simulink model "kif_halozat"  (R2020a)
settings: Solver=VariableStepAuto  StartTime=0.0  StopTime=10.0  RelTol=1e-3
libraries: powerlib x95, ee_lib x33
settings Model: Creator=Ákos  LastModifiedBy=Ákos

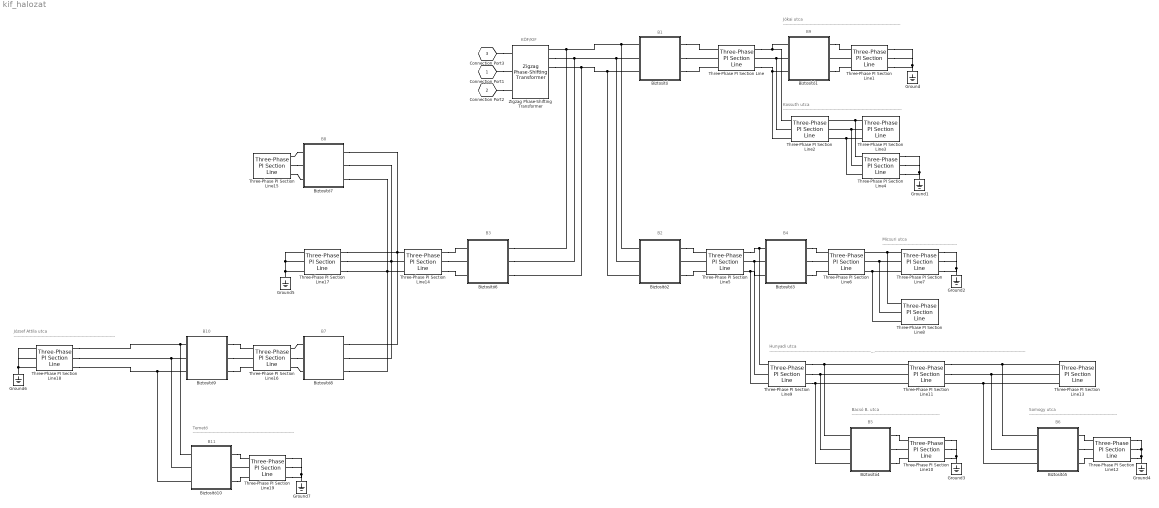
== system kif_halozat ==
  note: B2
  note: Jókai utca
      | ----------------------------------------------------------------------------------------
  note: B9
  note: B1
  note: KÖF/KIF
  note: Kossuth utca
      | -----------------------------------------------------------------------------------------
  note: B4
  note: Micsuri utca
      | --------------------------------------------------------
  note: B5
  note: B6
  note: Bacsó B. utca
      | ------------------------------------------------------------------
  note: Somogy utca
      | ------------------------------------------------------------------
  note: Hunyadi utca
      | -----------------------------------------------------------------------------------------------------------------------------------------------------------------------------------------------------------------------
  note: B3
  note: B8
  note: B7
  note: B10
  note: József Attila utca
      | ----------------------------------------------------------------------------
  note: B11
  note: Temető
      | ----------------------------------------------------------------------------
  Biztosító : Subsystem
  Biztosító1 : Subsystem
  Biztosító10 : Subsystem
  Biztosító2 : Subsystem
  Biztosító3 : Subsystem
  Biztosító4 : Subsystem
  Biztosító5 : Subsystem
  Biztosító6 : Subsystem
  Biztosító7 : Subsystem
  Biztosító8 : Subsystem
  Biztosító9 : Subsystem
  Ground{,1..7} (8 alike) : powerlib/Elements/Ground  LConnTagsString=a
  Three-Phase PI Section Line : powerlib/Elements/Three-Phase PI Section Line  LConnTagsString=a|b|c  RConnTagsString=A|B|C  Frequency=50  Resistances=[ 0.01273 0.3864]  Inductances="[ 0.9337e-3  4.1264e-3]"  Capacitances=[12.74e-9 7.751e-9]  Length=0.195
  Three-Phase PI Section Line1 : powerlib/Elements/Three-Phase PI Section Line  LConnTagsString=a|b|c  RConnTagsString=A|B|C  Frequency=50  Resistances=[ 0.01273 0.3864]  Inductances="[ 0.9337e-3  4.1264e-3]"  Capacitances=[12.74e-9 7.751e-9]  Length=0.3
  Three-Phase PI Section Line10 : powerlib/Elements/Three-Phase PI Section Line  LConnTagsString=a|b|c  RConnTagsString=A|B|C  Frequency=50  Resistances=[ 0.01273 0.3864]  Inductances="[ 0.9337e-3  4.1264e-3]"  Capacitances=[12.74e-9 7.751e-9]  Length=0.193
  Three-Phase PI Section Line11 : powerlib/Elements/Three-Phase PI Section Line  LConnTagsString=a|b|c  RConnTagsString=A|B|C  Frequency=50  Resistances=[ 0.01273 0.3864]  Inductances="[ 0.9337e-3  4.1264e-3]"  Capacitances=[12.74e-9 7.751e-9]  Length=0.151
  Three-Phase PI Section Line12 : powerlib/Elements/Three-Phase PI Section Line  LConnTagsString=a|b|c  RConnTagsString=A|B|C  Frequency=50  Resistances=[ 0.01273 0.3864]  Inductances="[ 0.9337e-3  4.1264e-3]"  Capacitances=[12.74e-9 7.751e-9]  Length=0.151
  Three-Phase PI Section Line13 : powerlib/Elements/Three-Phase PI Section Line  LConnTagsString=a|b|c  RConnTagsString=A|B|C  Frequency=50  Resistances=[ 0.01273 0.3864]  Inductances="[ 0.9337e-3  4.1264e-3]"  Capacitances=[12.74e-9 7.751e-9]  Length=0.151
  Three-Phase PI Section Line14 : powerlib/Elements/Three-Phase PI Section Line  LConnTagsString=a|b|c  RConnTagsString=A|B|C  Frequency=50  Resistances=[ 0.01273 0.3864]  Inductances="[ 0.9337e-3  4.1264e-3]"  Capacitances=[12.74e-9 7.751e-9]  Length=0.063
  Three-Phase PI Section Line15 : powerlib/Elements/Three-Phase PI Section Line  LConnTagsString=a|b|c  RConnTagsString=A|B|C  Frequency=50  Resistances=[ 0.01273 0.3864]  Inductances="[ 0.9337e-3  4.1264e-3]"  Capacitances=[12.74e-9 7.751e-9]  Length=0.010
  Three-Phase PI Section Line16 : powerlib/Elements/Three-Phase PI Section Line  LConnTagsString=a|b|c  RConnTagsString=A|B|C  Frequency=50  Resistances=[ 0.01273 0.3864]  Inductances="[ 0.9337e-3  4.1264e-3]"  Capacitances=[12.74e-9 7.751e-9]  Length=0.249
  Three-Phase PI Section Line17 : powerlib/Elements/Three-Phase PI Section Line  LConnTagsString=a|b|c  RConnTagsString=A|B|C  Frequency=50  Resistances=[ 0.01273 0.3864]  Inductances="[ 0.9337e-3  4.1264e-3]"  Capacitances=[12.74e-9 7.751e-9]  Length=0.217
  Three-Phase PI Section Line18 : powerlib/Elements/Three-Phase PI Section Line  LConnTagsString=a|b|c  RConnTagsString=A|B|C  Frequency=50  Resistances=[ 0.01273 0.3864]  Inductances="[ 0.9337e-3  4.1264e-3]"  Capacitances=[12.74e-9 7.751e-9]  Length=0.157
  Three-Phase PI Section Line19 : powerlib/Elements/Three-Phase PI Section Line  LConnTagsString=a|b|c  RConnTagsString=A|B|C  Frequency=50  Resistances=[ 0.01273 0.3864]  Inductances="[ 0.9337e-3  4.1264e-3]"  Capacitances=[12.74e-9 7.751e-9]  Length=0.187
  Three-Phase PI Section Line2 : powerlib/Elements/Three-Phase PI Section Line  LConnTagsString=a|b|c  RConnTagsString=A|B|C  Frequency=50  Resistances=[ 0.01273 0.3864]  Inductances="[ 0.9337e-3  4.1264e-3]"  Capacitances=[12.74e-9 7.751e-9]  Length=0.317
  Three-Phase PI Section Line3 : powerlib/Elements/Three-Phase PI Section Line  LConnTagsString=a|b|c  RConnTagsString=A|B|C  Frequency=50  Resistances=[ 0.01273 0.3864]  Inductances="[ 0.9337e-3  4.1264e-3]"  Capacitances=[12.74e-9 7.751e-9]  Length=0.078
  Three-Phase PI Section Line4 : powerlib/Elements/Three-Phase PI Section Line  LConnTagsString=a|b|c  RConnTagsString=A|B|C  Frequency=50  Resistances=[ 0.01273 0.3864]  Inductances="[ 0.9337e-3  4.1264e-3]"  Capacitances=[12.74e-9 7.751e-9]  Length=0.036
  Three-Phase PI Section Line5 : powerlib/Elements/Three-Phase PI Section Line  LConnTagsString=a|b|c  RConnTagsString=A|B|C  Frequency=50  Resistances=[ 0.01273 0.3864]  Inductances="[ 0.9337e-3  4.1264e-3]"  Capacitances=[12.74e-9 7.751e-9]  Length=0.070
  Three-Phase PI Section Line6 : powerlib/Elements/Three-Phase PI Section Line  LConnTagsString=a|b|c  RConnTagsString=A|B|C  Frequency=50  Resistances=[ 0.01273 0.3864]  Inductances="[ 0.9337e-3  4.1264e-3]"  Capacitances=[12.74e-9 7.751e-9]  Length=0.092
  Three-Phase PI Section Line7 : powerlib/Elements/Three-Phase PI Section Line  LConnTagsString=a|b|c  RConnTagsString=A|B|C  Frequency=50  Resistances=[ 0.01273 0.3864]  Inductances="[ 0.9337e-3  4.1264e-3]"  Capacitances=[12.74e-9 7.751e-9]  Length=0.270
  Three-Phase PI Section Line8 : powerlib/Elements/Three-Phase PI Section Line  LConnTagsString=a|b|c  RConnTagsString=A|B|C  Frequency=50  Resistances=[ 0.01273 0.3864]  Inductances="[ 0.9337e-3  4.1264e-3]"  Capacitances=[12.74e-9 7.751e-9]  Length=0.066
  Three-Phase PI Section Line9 : powerlib/Elements/Three-Phase PI Section Line  LConnTagsString=a|b|c  RConnTagsString=A|B|C  Frequency=50  Resistances=[ 0.01273 0.3864]  Inductances="[ 0.9337e-3  4.1264e-3]"  Capacitances=[12.74e-9 7.751e-9]  Length=0.106
  Zigzag Phase-Shifting Transformer : powerlib/Elements/Zigzag Phase-Shifting Transformer  SecondaryConnection=Y  SetSaturation=off  SetInitialFlux=off  Measurements=None  UNITS=SI  NominalPower=[ 120e3 50]  PrimaryVoltage=0.42e3  SecondaryVoltage="[ 21e3  +90]"  Winding1=[0.002488 0.00026399]  Winding2=[0.00017863 1.8954e-05]  Winding3=[0.018 0.0019099]  RmLm=[622.01 1.6499]  Rm=622.01  Saturation=[0 0;17.569 28.988;7320.5 36.718]  InitialFluxes=[0 0 0]  BreakLoop=off  DiscreteSolver=Trapezoidal iterative  DataType=on
      settings: SourceProductBaseCode=PS
  Connection Port1 : PMIOPort  Tag=PMCPort  Side=Left
  Connection Port2 : PMIOPort  Tag=PMCPort  Port=2  Side=Left
  Connection Port3 : PMIOPort  Tag=PMCPort  Port=3  Side=Left
  connections:
  Biztosító/RConn1 -- Three-Phase PI Section Line/LConn1
  Biztosító/LConn1 -- Biztosító2/LConn1 -- Biztosító6/LConn1 -- Zigzag Phase-Shifting Transformer/LConn1
  Biztosító/RConn2 -- Three-Phase PI Section Line/LConn2
  Zigzag Phase-Shifting Transformer/LConn2 -- Biztosító6/LConn2 -- Biztosító2/LConn2 -- Biztosító/LConn2
  Biztosító/RConn3 -- Three-Phase PI Section Line/LConn3
  Zigzag Phase-Shifting Transformer/LConn3 -- Biztosító6/LConn3 -- Biztosító2/LConn3 -- Biztosító/LConn3
  Biztosító1/LConn2 -- Three-Phase PI Section Line2/LConn2 -- Three-Phase PI Section Line/RConn2
  Three-Phase PI Section Line/RConn1 -- Three-Phase PI Section Line2/LConn1 -- Biztosító1/LConn1
  Three-Phase PI Section Line/RConn3 -- Three-Phase PI Section Line2/LConn3 -- Biztosító1/LConn3
  Three-Phase PI Section Line1/LConn2 -- Biztosító1/RConn2
  Biztosító1/RConn1 -- Three-Phase PI Section Line1/LConn1
  Biztosító1/RConn3 -- Three-Phase PI Section Line1/LConn3
  Three-Phase PI Section Line1/RConn3 -- Three-Phase PI Section Line1/RConn1 -- Three-Phase PI Section Line1/RConn2 -- Ground/LConn1
  Three-Phase PI Section Line3/LConn1 -- Three-Phase PI Section Line4/LConn1 -- Three-Phase PI Section Line2/RConn1
  Three-Phase PI Section Line3/LConn2 -- Three-Phase PI Section Line4/LConn2 -- Three-Phase PI Section Line2/RConn2
  Three-Phase PI Section Line3/LConn3 -- Three-Phase PI Section Line4/LConn3 -- Three-Phase PI Section Line2/RConn3
  Three-Phase PI Section Line4/RConn1 -- Three-Phase PI Section Line4/RConn2 -- Three-Phase PI Section Line4/RConn3 -- Ground1/LConn1
  Three-Phase PI Section Line5/LConn2 -- Biztosító2/RConn2
  Biztosító2/RConn1 -- Three-Phase PI Section Line5/LConn1
  Biztosító2/RConn3 -- Three-Phase PI Section Line5/LConn3
  Biztosító3/LConn2 -- Three-Phase PI Section Line9/LConn2 -- Three-Phase PI Section Line5/RConn2
  Three-Phase PI Section Line5/RConn1 -- Three-Phase PI Section Line9/LConn1 -- Biztosító3/LConn1
  Three-Phase PI Section Line5/RConn3 -- Three-Phase PI Section Line9/LConn3 -- Biztosító3/LConn3
  Biztosító3/RConn1 -- Three-Phase PI Section Line6/LConn1
  Biztosító3/RConn2 -- Three-Phase PI Section Line6/LConn2
  Biztosító3/RConn3 -- Three-Phase PI Section Line6/LConn3
  Three-Phase PI Section Line7/LConn1 -- Three-Phase PI Section Line8/LConn1 -- Three-Phase PI Section Line6/RConn1
  Three-Phase PI Section Line7/LConn2 -- Three-Phase PI Section Line8/LConn2 -- Three-Phase PI Section Line6/RConn2
  Three-Phase PI Section Line7/LConn3 -- Three-Phase PI Section Line8/LConn3 -- Three-Phase PI Section Line6/RConn3
  Ground2/LConn1 -- Three-Phase PI Section Line7/RConn3 -- Three-Phase PI Section Line7/RConn1 -- Three-Phase PI Section Line7/RConn2
  Three-Phase PI Section Line9/RConn1 -- Three-Phase PI Section Line11/LConn1 -- Biztosító4/LConn1
  Three-Phase PI Section Line9/RConn2 -- Three-Phase PI Section Line11/LConn2 -- Biztosító4/LConn2
  Three-Phase PI Section Line9/RConn3 -- Three-Phase PI Section Line11/LConn3 -- Biztosító4/LConn3
  Biztosító4/RConn1 -- Three-Phase PI Section Line10/LConn1
  Biztosító4/RConn2 -- Three-Phase PI Section Line10/LConn2
  Biztosító4/RConn3 -- Three-Phase PI Section Line10/LConn3
  Ground3/LConn1 -- Three-Phase PI Section Line10/RConn3 -- Three-Phase PI Section Line10/RConn1 -- Three-Phase PI Section Line10/RConn2
  Three-Phase PI Section Line11/RConn1 -- Three-Phase PI Section Line13/LConn1 -- Biztosító5/LConn1
  Three-Phase PI Section Line11/RConn2 -- Three-Phase PI Section Line13/LConn2 -- Biztosító5/LConn2
  Biztosító5/LConn3 -- Three-Phase PI Section Line13/LConn3 -- Three-Phase PI Section Line11/RConn3
  Three-Phase PI Section Line12/RConn1 -- Three-Phase PI Section Line12/RConn2 -- Three-Phase PI Section Line12/RConn3 -- Ground4/LConn1
  Biztosító5/RConn3 -- Three-Phase PI Section Line12/LConn3
  Biztosító5/RConn2 -- Three-Phase PI Section Line12/LConn2
  Biztosító5/RConn1 -- Three-Phase PI Section Line12/LConn1
  Three-Phase PI Section Line14/RConn1 -- Biztosító6/RConn1
  Three-Phase PI Section Line14/RConn2 -- Biztosító6/RConn2
  Three-Phase PI Section Line14/RConn3 -- Biztosító6/RConn3
  Biztosító7/RConn1 -- Three-Phase PI Section Line15/RConn1
  Three-Phase PI Section Line15/RConn2 -- Biztosító7/RConn2
  Three-Phase PI Section Line15/RConn3 -- Biztosító7/RConn3
  Three-Phase PI Section Line16/RConn3 -- Biztosító8/RConn3
  Three-Phase PI Section Line16/RConn2 -- Biztosító8/RConn2
  Biztosító8/RConn1 -- Three-Phase PI Section Line16/RConn1
  Three-Phase PI Section Line17/RConn1 -- Biztosító8/LConn1 -- Biztosító7/LConn1 -- Three-Phase PI Section Line14/LConn1
  Three-Phase PI Section Line17/RConn2 -- Biztosító8/LConn2 -- Biztosító7/LConn2 -- Three-Phase PI Section Line14/LConn2
  Three-Phase PI Section Line17/RConn3 -- Biztosító8/LConn3 -- Biztosító7/LConn3 -- Three-Phase PI Section Line14/LConn3
  Three-Phase PI Section Line17/LConn1 -- Three-Phase PI Section Line17/LConn2 -- Three-Phase PI Section Line17/LConn3 -- Ground5/LConn1
  Biztosító9/LConn2 -- Three-Phase PI Section Line16/LConn2
  Biztosító9/LConn1 -- Three-Phase PI Section Line16/LConn1
  Biztosító9/LConn3 -- Three-Phase PI Section Line16/LConn3
  Three-Phase PI Section Line18/LConn3 -- Three-Phase PI Section Line18/LConn1 -- Three-Phase PI Section Line18/LConn2 -- Ground6/LConn1
  Three-Phase PI Section Line18/RConn2 -- Biztosító10/LConn2 -- Biztosító9/RConn2
  Three-Phase PI Section Line18/RConn1 -- Biztosító10/LConn1 -- Biztosító9/RConn1
  Three-Phase PI Section Line18/RConn3 -- Biztosító10/LConn3 -- Biztosító9/RConn3
  Three-Phase PI Section Line19/LConn2 -- Biztosító10/RConn2
  Biztosító10/RConn1 -- Three-Phase PI Section Line19/LConn1
  Biztosító10/RConn3 -- Three-Phase PI Section Line19/LConn3
  Three-Phase PI Section Line19/RConn1 -- Three-Phase PI Section Line19/RConn2 -- Three-Phase PI Section Line19/RConn3 -- Ground7/LConn1
  Connection Port1/RConn1 -- Zigzag Phase-Shifting Transformer/RConn2
  Connection Port2/RConn1 -- Zigzag Phase-Shifting Transformer/RConn3
  Connection Port3/RConn1 -- Zigzag Phase-Shifting Transformer/RConn1

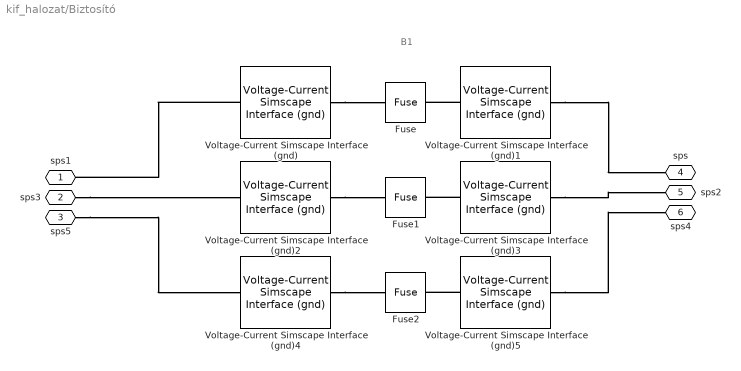
== system kif_halozat/Biztosító ==
  note: B1
  Fuse : ee_lib/Switches & Breakers/Fuse  prm=1  I_rated=125 A  melt_margin=1  T_fuse=0 s  I2t=1 s*A^2  I_vec=[1.9, 2, 2.5, 30] A  t_vec=[10000, 1, .3, .001] s  R_closed=0.01 Ohm  G_open=1e-8 1/Ohm  exposemeasurement=ee.enum.exposemeasurement.hidden
      settings: SourceProductBaseCode=PS  InternalSimscapePortConfiguration="{\"Bottom\":[],\"Left\":[{\"id\":\"p\",\"label\":\"\",\"type\":\"foundation.electrical.electrical\"}],\"Right\":[{\"id\":\"n\",\"label\":\"\",\"type\":\"foundation.electrical.electrical\"}],\"Top\":[]}"
  Fuse1 : ee_lib/Switches & Breakers/Fuse  prm=1  I_rated=125 A  melt_margin=1  T_fuse=0 s  I2t=1 s*A^2  I_vec=[1.9, 2, 2.5, 30] A  t_vec=[10000, 1, .3, .001] s  R_closed=0.01 Ohm  G_open=1e-8 1/Ohm  exposemeasurement=ee.enum.exposemeasurement.hidden
      settings: SourceProductBaseCode=PS  InternalSimscapePortConfiguration="{\"Bottom\":[],\"Left\":[{\"id\":\"p\",\"label\":\"\",\"type\":\"foundation.electrical.electrical\"}],\"Right\":[{\"id\":\"n\",\"label\":\"\",\"type\":\"foundation.electrical.electrical\"}],\"Top\":[]}"
  Fuse2 : ee_lib/Switches & Breakers/Fuse  prm=1  I_rated=125 A  melt_margin=1  T_fuse=0 s  I2t=1 s*A^2  I_vec=[1.9, 2, 2.5, 30] A  t_vec=[10000, 1, .3, .001] s  R_closed=0.01 Ohm  G_open=1e-8 1/Ohm  exposemeasurement=ee.enum.exposemeasurement.hidden
      settings: SourceProductBaseCode=PS  InternalSimscapePortConfiguration="{\"Bottom\":[],\"Left\":[{\"id\":\"p\",\"label\":\"\",\"type\":\"foundation.electrical.electrical\"}],\"Right\":[{\"id\":\"n\",\"label\":\"\",\"type\":\"foundation.electrical.electrical\"}],\"Top\":[]}"
  Voltage-Current Simscape Interface (gnd){,1..5} (6 alike) : powerlib/Interface Elements/Voltage-Current Simscape Interface (gnd)  DFT=off  Fmode=Low pass filter (continuous)  T=1e-6  Ts=50e-6  i0=0  v0=0  Sd=Specialized Power Systems side  Measurements=off
      settings: SourceProductBaseCode=PS
  sps1 : PMIOPort  Side=Left
  sps3 : PMIOPort  Port=2  Side=Left
  sps5 : PMIOPort  Port=3  Side=Left
  sps : PMIOPort  Port=4  Side=Right
  sps2 : PMIOPort  Port=5  Side=Right
  sps4 : PMIOPort  Port=6  Side=Right
  connections:
  Voltage-Current Simscape Interface (gnd)5/RConn1 -- Fuse2/RConn1
  Voltage-Current Simscape Interface (gnd)4/RConn1 -- Fuse2/LConn1
  sps3/RConn1 -- Voltage-Current Simscape Interface (gnd)2/LConn1
  Voltage-Current Simscape Interface (gnd)/RConn1 -- Fuse/LConn1
  Voltage-Current Simscape Interface (gnd)/LConn1 -- sps1/RConn1
  Voltage-Current Simscape Interface (gnd)1/RConn1 -- Fuse/RConn1
  Voltage-Current Simscape Interface (gnd)2/RConn1 -- Fuse1/LConn1
  sps5/RConn1 -- Voltage-Current Simscape Interface (gnd)4/LConn1
  Voltage-Current Simscape Interface (gnd)5/LConn1 -- sps4/RConn1
  Voltage-Current Simscape Interface (gnd)3/RConn1 -- Fuse1/RConn1
  Voltage-Current Simscape Interface (gnd)1/LConn1 -- sps/RConn1
  Voltage-Current Simscape Interface (gnd)3/LConn1 -- sps2/RConn1

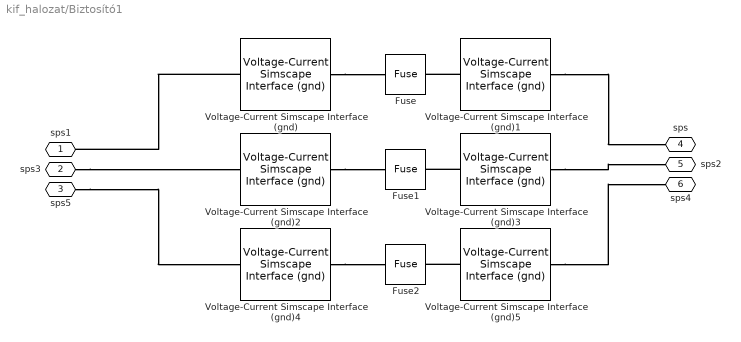
== system kif_halozat/Biztosító1 ==
  Fuse : ee_lib/Switches & Breakers/Fuse  prm=1  I_rated=80 A  melt_margin=1  T_fuse=0 s  I2t=1 s*A^2  I_vec=[1.9, 2, 2.5, 30] A  t_vec=[10000, 1, .3, .001] s  R_closed=0.01 Ohm  G_open=1e-8 1/Ohm  exposemeasurement=ee.enum.exposemeasurement.hidden
      settings: SourceProductBaseCode=PS  InternalSimscapePortConfiguration="{\"Bottom\":[],\"Left\":[{\"id\":\"p\",\"label\":\"\",\"type\":\"foundation.electrical.electrical\"}],\"Right\":[{\"id\":\"n\",\"label\":\"\",\"type\":\"foundation.electrical.electrical\"}],\"Top\":[]}"
  Fuse1 : ee_lib/Switches & Breakers/Fuse  prm=1  I_rated=80 A  melt_margin=1  T_fuse=0 s  I2t=1 s*A^2  I_vec=[1.9, 2, 2.5, 30] A  t_vec=[10000, 1, .3, .001] s  R_closed=0.01 Ohm  G_open=1e-8 1/Ohm  exposemeasurement=ee.enum.exposemeasurement.hidden
      settings: SourceProductBaseCode=PS  InternalSimscapePortConfiguration="{\"Bottom\":[],\"Left\":[{\"id\":\"p\",\"label\":\"\",\"type\":\"foundation.electrical.electrical\"}],\"Right\":[{\"id\":\"n\",\"label\":\"\",\"type\":\"foundation.electrical.electrical\"}],\"Top\":[]}"
  Fuse2 : ee_lib/Switches & Breakers/Fuse  prm=1  I_rated=80 A  melt_margin=1  T_fuse=0 s  I2t=1 s*A^2  I_vec=[1.9, 2, 2.5, 30] A  t_vec=[10000, 1, .3, .001] s  R_closed=0.01 Ohm  G_open=1e-8 1/Ohm  exposemeasurement=ee.enum.exposemeasurement.hidden
      settings: SourceProductBaseCode=PS  InternalSimscapePortConfiguration="{\"Bottom\":[],\"Left\":[{\"id\":\"p\",\"label\":\"\",\"type\":\"foundation.electrical.electrical\"}],\"Right\":[{\"id\":\"n\",\"label\":\"\",\"type\":\"foundation.electrical.electrical\"}],\"Top\":[]}"
  Voltage-Current Simscape Interface (gnd){,1..5} (6 alike) : powerlib/Interface Elements/Voltage-Current Simscape Interface (gnd)  DFT=off  Fmode=Low pass filter (continuous)  T=1e-6  Ts=50e-6  i0=0  v0=0  Sd=Specialized Power Systems side  Measurements=off
      settings: SourceProductBaseCode=PS
  sps1 : PMIOPort  Side=Left
  sps3 : PMIOPort  Port=2  Side=Left
  sps5 : PMIOPort  Port=3  Side=Left
  sps : PMIOPort  Port=4  Side=Right
  sps2 : PMIOPort  Port=5  Side=Right
  sps4 : PMIOPort  Port=6  Side=Right
  connections:
  Voltage-Current Simscape Interface (gnd)3/LConn1 -- sps2/RConn1
  Voltage-Current Simscape Interface (gnd)1/LConn1 -- sps/RConn1
  Voltage-Current Simscape Interface (gnd)3/RConn1 -- Fuse1/RConn1
  Voltage-Current Simscape Interface (gnd)5/LConn1 -- sps4/RConn1
  sps5/RConn1 -- Voltage-Current Simscape Interface (gnd)4/LConn1
  Voltage-Current Simscape Interface (gnd)2/RConn1 -- Fuse1/LConn1
  Voltage-Current Simscape Interface (gnd)1/RConn1 -- Fuse/RConn1
  Voltage-Current Simscape Interface (gnd)/LConn1 -- sps1/RConn1
  Voltage-Current Simscape Interface (gnd)/RConn1 -- Fuse/LConn1
  sps3/RConn1 -- Voltage-Current Simscape Interface (gnd)2/LConn1
  Voltage-Current Simscape Interface (gnd)4/RConn1 -- Fuse2/LConn1
  Voltage-Current Simscape Interface (gnd)5/RConn1 -- Fuse2/RConn1

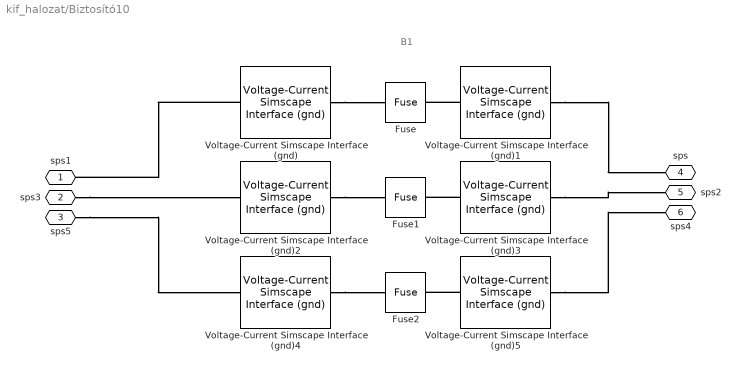
== system kif_halozat/Biztosító10 ==
  note: B1
  Fuse : ee_lib/Switches & Breakers/Fuse  prm=1  I_rated=125 A  melt_margin=1  T_fuse=0 s  I2t=1 s*A^2  I_vec=[1.9, 2, 2.5, 30] A  t_vec=[10000, 1, .3, .001] s  R_closed=0.01 Ohm  G_open=1e-8 1/Ohm  exposemeasurement=ee.enum.exposemeasurement.hidden
      settings: SourceProductBaseCode=PS  InternalSimscapePortConfiguration="{\"Bottom\":[],\"Left\":[{\"id\":\"p\",\"label\":\"\",\"type\":\"foundation.electrical.electrical\"}],\"Right\":[{\"id\":\"n\",\"label\":\"\",\"type\":\"foundation.electrical.electrical\"}],\"Top\":[]}"
  Fuse1 : ee_lib/Switches & Breakers/Fuse  prm=1  I_rated=125 A  melt_margin=1  T_fuse=0 s  I2t=1 s*A^2  I_vec=[1.9, 2, 2.5, 30] A  t_vec=[10000, 1, .3, .001] s  R_closed=0.01 Ohm  G_open=1e-8 1/Ohm  exposemeasurement=ee.enum.exposemeasurement.hidden
      settings: SourceProductBaseCode=PS  InternalSimscapePortConfiguration="{\"Bottom\":[],\"Left\":[{\"id\":\"p\",\"label\":\"\",\"type\":\"foundation.electrical.electrical\"}],\"Right\":[{\"id\":\"n\",\"label\":\"\",\"type\":\"foundation.electrical.electrical\"}],\"Top\":[]}"
  Fuse2 : ee_lib/Switches & Breakers/Fuse  prm=1  I_rated=125 A  melt_margin=1  T_fuse=0 s  I2t=1 s*A^2  I_vec=[1.9, 2, 2.5, 30] A  t_vec=[10000, 1, .3, .001] s  R_closed=0.01 Ohm  G_open=1e-8 1/Ohm  exposemeasurement=ee.enum.exposemeasurement.hidden
      settings: SourceProductBaseCode=PS  InternalSimscapePortConfiguration="{\"Bottom\":[],\"Left\":[{\"id\":\"p\",\"label\":\"\",\"type\":\"foundation.electrical.electrical\"}],\"Right\":[{\"id\":\"n\",\"label\":\"\",\"type\":\"foundation.electrical.electrical\"}],\"Top\":[]}"
  Voltage-Current Simscape Interface (gnd){,1..5} (6 alike) : powerlib/Interface Elements/Voltage-Current Simscape Interface (gnd)  DFT=off  Fmode=Low pass filter (continuous)  T=1e-6  Ts=50e-6  i0=0  v0=0  Sd=Specialized Power Systems side  Measurements=off
      settings: SourceProductBaseCode=PS
  sps1 : PMIOPort  Side=Left
  sps3 : PMIOPort  Port=2  Side=Left
  sps5 : PMIOPort  Port=3  Side=Left
  sps : PMIOPort  Port=4  Side=Right
  sps2 : PMIOPort  Port=5  Side=Right
  sps4 : PMIOPort  Port=6  Side=Right
  connections:
  Voltage-Current Simscape Interface (gnd)5/RConn1 -- Fuse2/RConn1
  Voltage-Current Simscape Interface (gnd)4/RConn1 -- Fuse2/LConn1
  sps3/RConn1 -- Voltage-Current Simscape Interface (gnd)2/LConn1
  Voltage-Current Simscape Interface (gnd)/RConn1 -- Fuse/LConn1
  Voltage-Current Simscape Interface (gnd)/LConn1 -- sps1/RConn1
  Voltage-Current Simscape Interface (gnd)1/RConn1 -- Fuse/RConn1
  Voltage-Current Simscape Interface (gnd)2/RConn1 -- Fuse1/LConn1
  sps5/RConn1 -- Voltage-Current Simscape Interface (gnd)4/LConn1
  Voltage-Current Simscape Interface (gnd)5/LConn1 -- sps4/RConn1
  Voltage-Current Simscape Interface (gnd)3/RConn1 -- Fuse1/RConn1
  Voltage-Current Simscape Interface (gnd)1/LConn1 -- sps/RConn1
  Voltage-Current Simscape Interface (gnd)3/LConn1 -- sps2/RConn1

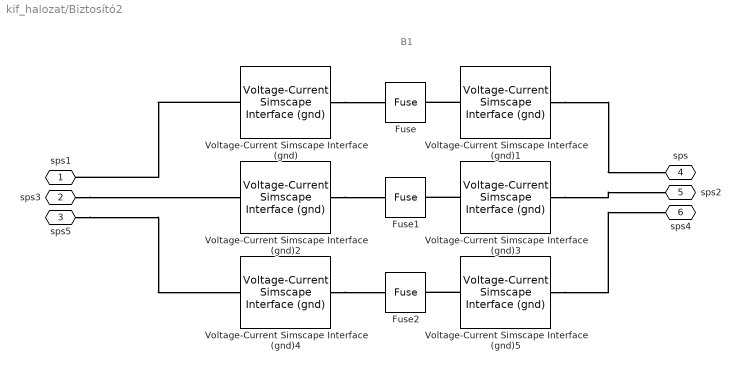
== system kif_halozat/Biztosító2 ==
  note: B1
  Fuse : ee_lib/Switches & Breakers/Fuse  prm=1  I_rated=125 A  melt_margin=1  T_fuse=0 s  I2t=1 s*A^2  I_vec=[1.9, 2, 2.5, 30] A  t_vec=[10000, 1, .3, .001] s  R_closed=0.01 Ohm  G_open=1e-8 1/Ohm  exposemeasurement=ee.enum.exposemeasurement.hidden
      settings: SourceProductBaseCode=PS  InternalSimscapePortConfiguration="{\"Bottom\":[],\"Left\":[{\"id\":\"p\",\"label\":\"\",\"type\":\"foundation.electrical.electrical\"}],\"Right\":[{\"id\":\"n\",\"label\":\"\",\"type\":\"foundation.electrical.electrical\"}],\"Top\":[]}"
  Fuse1 : ee_lib/Switches & Breakers/Fuse  prm=1  I_rated=125 A  melt_margin=1  T_fuse=0 s  I2t=1 s*A^2  I_vec=[1.9, 2, 2.5, 30] A  t_vec=[10000, 1, .3, .001] s  R_closed=0.01 Ohm  G_open=1e-8 1/Ohm  exposemeasurement=ee.enum.exposemeasurement.hidden
      settings: SourceProductBaseCode=PS  InternalSimscapePortConfiguration="{\"Bottom\":[],\"Left\":[{\"id\":\"p\",\"label\":\"\",\"type\":\"foundation.electrical.electrical\"}],\"Right\":[{\"id\":\"n\",\"label\":\"\",\"type\":\"foundation.electrical.electrical\"}],\"Top\":[]}"
  Fuse2 : ee_lib/Switches & Breakers/Fuse  prm=1  I_rated=125 A  melt_margin=1  T_fuse=0 s  I2t=1 s*A^2  I_vec=[1.9, 2, 2.5, 30] A  t_vec=[10000, 1, .3, .001] s  R_closed=0.01 Ohm  G_open=1e-8 1/Ohm  exposemeasurement=ee.enum.exposemeasurement.hidden
      settings: SourceProductBaseCode=PS  InternalSimscapePortConfiguration="{\"Bottom\":[],\"Left\":[{\"id\":\"p\",\"label\":\"\",\"type\":\"foundation.electrical.electrical\"}],\"Right\":[{\"id\":\"n\",\"label\":\"\",\"type\":\"foundation.electrical.electrical\"}],\"Top\":[]}"
  Voltage-Current Simscape Interface (gnd){,1..5} (6 alike) : powerlib/Interface Elements/Voltage-Current Simscape Interface (gnd)  DFT=off  Fmode=Low pass filter (continuous)  T=1e-6  Ts=50e-6  i0=0  v0=0  Sd=Specialized Power Systems side  Measurements=off
      settings: SourceProductBaseCode=PS
  sps1 : PMIOPort  Side=Left
  sps3 : PMIOPort  Port=2  Side=Left
  sps5 : PMIOPort  Port=3  Side=Left
  sps : PMIOPort  Port=4  Side=Right
  sps2 : PMIOPort  Port=5  Side=Right
  sps4 : PMIOPort  Port=6  Side=Right
  connections:
  Voltage-Current Simscape Interface (gnd)3/LConn1 -- sps2/RConn1
  Voltage-Current Simscape Interface (gnd)1/LConn1 -- sps/RConn1
  Voltage-Current Simscape Interface (gnd)3/RConn1 -- Fuse1/RConn1
  Voltage-Current Simscape Interface (gnd)5/LConn1 -- sps4/RConn1
  sps5/RConn1 -- Voltage-Current Simscape Interface (gnd)4/LConn1
  Voltage-Current Simscape Interface (gnd)2/RConn1 -- Fuse1/LConn1
  Voltage-Current Simscape Interface (gnd)1/RConn1 -- Fuse/RConn1
  Voltage-Current Simscape Interface (gnd)/LConn1 -- sps1/RConn1
  Voltage-Current Simscape Interface (gnd)/RConn1 -- Fuse/LConn1
  sps3/RConn1 -- Voltage-Current Simscape Interface (gnd)2/LConn1
  Voltage-Current Simscape Interface (gnd)4/RConn1 -- Fuse2/LConn1
  Voltage-Current Simscape Interface (gnd)5/RConn1 -- Fuse2/RConn1

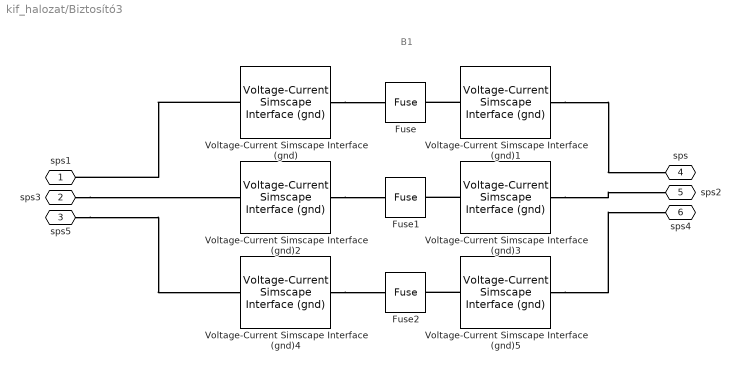
== system kif_halozat/Biztosító3 ==
  note: B1
  Fuse : ee_lib/Switches & Breakers/Fuse  prm=1  I_rated=125 A  melt_margin=1  T_fuse=0 s  I2t=1 s*A^2  I_vec=[1.9, 2, 2.5, 30] A  t_vec=[10000, 1, .3, .001] s  R_closed=0.01 Ohm  G_open=1e-8 1/Ohm  exposemeasurement=ee.enum.exposemeasurement.hidden
      settings: SourceProductBaseCode=PS  InternalSimscapePortConfiguration="{\"Bottom\":[],\"Left\":[{\"id\":\"p\",\"label\":\"\",\"type\":\"foundation.electrical.electrical\"}],\"Right\":[{\"id\":\"n\",\"label\":\"\",\"type\":\"foundation.electrical.electrical\"}],\"Top\":[]}"
  Fuse1 : ee_lib/Switches & Breakers/Fuse  prm=1  I_rated=125 A  melt_margin=1  T_fuse=0 s  I2t=1 s*A^2  I_vec=[1.9, 2, 2.5, 30] A  t_vec=[10000, 1, .3, .001] s  R_closed=0.01 Ohm  G_open=1e-8 1/Ohm  exposemeasurement=ee.enum.exposemeasurement.hidden
      settings: SourceProductBaseCode=PS  InternalSimscapePortConfiguration="{\"Bottom\":[],\"Left\":[{\"id\":\"p\",\"label\":\"\",\"type\":\"foundation.electrical.electrical\"}],\"Right\":[{\"id\":\"n\",\"label\":\"\",\"type\":\"foundation.electrical.electrical\"}],\"Top\":[]}"
  Fuse2 : ee_lib/Switches & Breakers/Fuse  prm=1  I_rated=125 A  melt_margin=1  T_fuse=0 s  I2t=1 s*A^2  I_vec=[1.9, 2, 2.5, 30] A  t_vec=[10000, 1, .3, .001] s  R_closed=0.01 Ohm  G_open=1e-8 1/Ohm  exposemeasurement=ee.enum.exposemeasurement.hidden
      settings: SourceProductBaseCode=PS  InternalSimscapePortConfiguration="{\"Bottom\":[],\"Left\":[{\"id\":\"p\",\"label\":\"\",\"type\":\"foundation.electrical.electrical\"}],\"Right\":[{\"id\":\"n\",\"label\":\"\",\"type\":\"foundation.electrical.electrical\"}],\"Top\":[]}"
  Voltage-Current Simscape Interface (gnd){,1..5} (6 alike) : powerlib/Interface Elements/Voltage-Current Simscape Interface (gnd)  DFT=off  Fmode=Low pass filter (continuous)  T=1e-6  Ts=50e-6  i0=0  v0=0  Sd=Specialized Power Systems side  Measurements=off
      settings: SourceProductBaseCode=PS
  sps1 : PMIOPort  Side=Left
  sps3 : PMIOPort  Port=2  Side=Left
  sps5 : PMIOPort  Port=3  Side=Left
  sps : PMIOPort  Port=4  Side=Right
  sps2 : PMIOPort  Port=5  Side=Right
  sps4 : PMIOPort  Port=6  Side=Right
  connections:
  Voltage-Current Simscape Interface (gnd)5/RConn1 -- Fuse2/RConn1
  Voltage-Current Simscape Interface (gnd)4/RConn1 -- Fuse2/LConn1
  sps3/RConn1 -- Voltage-Current Simscape Interface (gnd)2/LConn1
  Voltage-Current Simscape Interface (gnd)/RConn1 -- Fuse/LConn1
  Voltage-Current Simscape Interface (gnd)/LConn1 -- sps1/RConn1
  Voltage-Current Simscape Interface (gnd)1/RConn1 -- Fuse/RConn1
  Voltage-Current Simscape Interface (gnd)2/RConn1 -- Fuse1/LConn1
  sps5/RConn1 -- Voltage-Current Simscape Interface (gnd)4/LConn1
  Voltage-Current Simscape Interface (gnd)5/LConn1 -- sps4/RConn1
  Voltage-Current Simscape Interface (gnd)3/RConn1 -- Fuse1/RConn1
  Voltage-Current Simscape Interface (gnd)1/LConn1 -- sps/RConn1
  Voltage-Current Simscape Interface (gnd)3/LConn1 -- sps2/RConn1

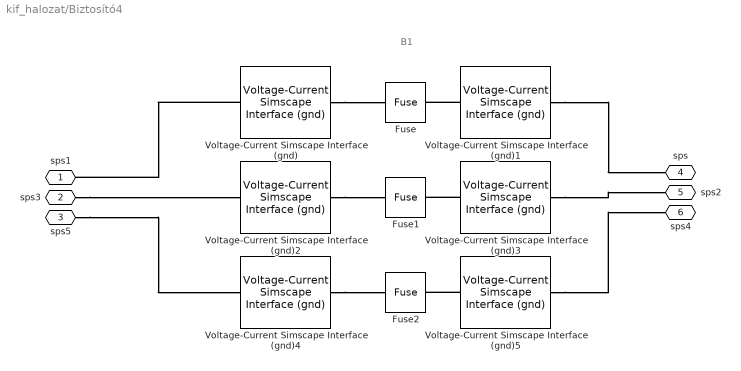
== system kif_halozat/Biztosító4 ==
  note: B1
  Fuse : ee_lib/Switches & Breakers/Fuse  prm=1  I_rated=125 A  melt_margin=1  T_fuse=0 s  I2t=1 s*A^2  I_vec=[1.9, 2, 2.5, 30] A  t_vec=[10000, 1, .3, .001] s  R_closed=0.01 Ohm  G_open=1e-8 1/Ohm  exposemeasurement=ee.enum.exposemeasurement.hidden
      settings: SourceProductBaseCode=PS  InternalSimscapePortConfiguration="{\"Bottom\":[],\"Left\":[{\"id\":\"p\",\"label\":\"\",\"type\":\"foundation.electrical.electrical\"}],\"Right\":[{\"id\":\"n\",\"label\":\"\",\"type\":\"foundation.electrical.electrical\"}],\"Top\":[]}"
  Fuse1 : ee_lib/Switches & Breakers/Fuse  prm=1  I_rated=125 A  melt_margin=1  T_fuse=0 s  I2t=1 s*A^2  I_vec=[1.9, 2, 2.5, 30] A  t_vec=[10000, 1, .3, .001] s  R_closed=0.01 Ohm  G_open=1e-8 1/Ohm  exposemeasurement=ee.enum.exposemeasurement.hidden
      settings: SourceProductBaseCode=PS  InternalSimscapePortConfiguration="{\"Bottom\":[],\"Left\":[{\"id\":\"p\",\"label\":\"\",\"type\":\"foundation.electrical.electrical\"}],\"Right\":[{\"id\":\"n\",\"label\":\"\",\"type\":\"foundation.electrical.electrical\"}],\"Top\":[]}"
  Fuse2 : ee_lib/Switches & Breakers/Fuse  prm=1  I_rated=125 A  melt_margin=1  T_fuse=0 s  I2t=1 s*A^2  I_vec=[1.9, 2, 2.5, 30] A  t_vec=[10000, 1, .3, .001] s  R_closed=0.01 Ohm  G_open=1e-8 1/Ohm  exposemeasurement=ee.enum.exposemeasurement.hidden
      settings: SourceProductBaseCode=PS  InternalSimscapePortConfiguration="{\"Bottom\":[],\"Left\":[{\"id\":\"p\",\"label\":\"\",\"type\":\"foundation.electrical.electrical\"}],\"Right\":[{\"id\":\"n\",\"label\":\"\",\"type\":\"foundation.electrical.electrical\"}],\"Top\":[]}"
  Voltage-Current Simscape Interface (gnd){,1..5} (6 alike) : powerlib/Interface Elements/Voltage-Current Simscape Interface (gnd)  DFT=off  Fmode=Low pass filter (continuous)  T=1e-6  Ts=50e-6  i0=0  v0=0  Sd=Specialized Power Systems side  Measurements=off
      settings: SourceProductBaseCode=PS
  sps1 : PMIOPort  Side=Left
  sps3 : PMIOPort  Port=2  Side=Left
  sps5 : PMIOPort  Port=3  Side=Left
  sps : PMIOPort  Port=4  Side=Right
  sps2 : PMIOPort  Port=5  Side=Right
  sps4 : PMIOPort  Port=6  Side=Right
  connections:
  Voltage-Current Simscape Interface (gnd)3/LConn1 -- sps2/RConn1
  Voltage-Current Simscape Interface (gnd)1/LConn1 -- sps/RConn1
  Voltage-Current Simscape Interface (gnd)3/RConn1 -- Fuse1/RConn1
  Voltage-Current Simscape Interface (gnd)5/LConn1 -- sps4/RConn1
  sps5/RConn1 -- Voltage-Current Simscape Interface (gnd)4/LConn1
  Voltage-Current Simscape Interface (gnd)2/RConn1 -- Fuse1/LConn1
  Voltage-Current Simscape Interface (gnd)1/RConn1 -- Fuse/RConn1
  Voltage-Current Simscape Interface (gnd)/LConn1 -- sps1/RConn1
  Voltage-Current Simscape Interface (gnd)/RConn1 -- Fuse/LConn1
  sps3/RConn1 -- Voltage-Current Simscape Interface (gnd)2/LConn1
  Voltage-Current Simscape Interface (gnd)4/RConn1 -- Fuse2/LConn1
  Voltage-Current Simscape Interface (gnd)5/RConn1 -- Fuse2/RConn1

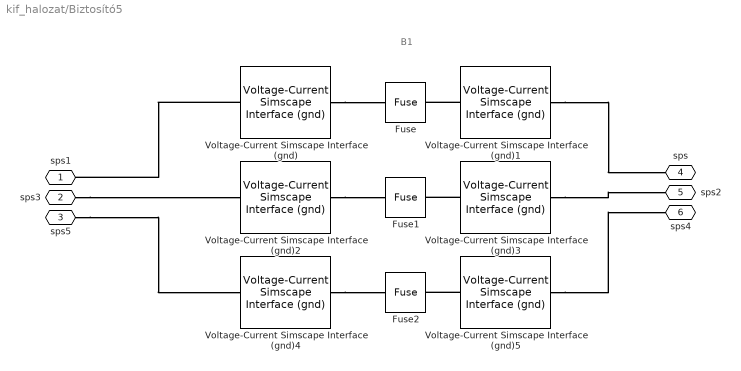
== system kif_halozat/Biztosító5 ==
  note: B1
  Fuse : ee_lib/Switches & Breakers/Fuse  prm=1  I_rated=125 A  melt_margin=1  T_fuse=0 s  I2t=1 s*A^2  I_vec=[1.9, 2, 2.5, 30] A  t_vec=[10000, 1, .3, .001] s  R_closed=0.01 Ohm  G_open=1e-8 1/Ohm  exposemeasurement=ee.enum.exposemeasurement.hidden
      settings: SourceProductBaseCode=PS  InternalSimscapePortConfiguration="{\"Bottom\":[],\"Left\":[{\"id\":\"p\",\"label\":\"\",\"type\":\"foundation.electrical.electrical\"}],\"Right\":[{\"id\":\"n\",\"label\":\"\",\"type\":\"foundation.electrical.electrical\"}],\"Top\":[]}"
  Fuse1 : ee_lib/Switches & Breakers/Fuse  prm=1  I_rated=125 A  melt_margin=1  T_fuse=0 s  I2t=1 s*A^2  I_vec=[1.9, 2, 2.5, 30] A  t_vec=[10000, 1, .3, .001] s  R_closed=0.01 Ohm  G_open=1e-8 1/Ohm  exposemeasurement=ee.enum.exposemeasurement.hidden
      settings: SourceProductBaseCode=PS  InternalSimscapePortConfiguration="{\"Bottom\":[],\"Left\":[{\"id\":\"p\",\"label\":\"\",\"type\":\"foundation.electrical.electrical\"}],\"Right\":[{\"id\":\"n\",\"label\":\"\",\"type\":\"foundation.electrical.electrical\"}],\"Top\":[]}"
  Fuse2 : ee_lib/Switches & Breakers/Fuse  prm=1  I_rated=125 A  melt_margin=1  T_fuse=0 s  I2t=1 s*A^2  I_vec=[1.9, 2, 2.5, 30] A  t_vec=[10000, 1, .3, .001] s  R_closed=0.01 Ohm  G_open=1e-8 1/Ohm  exposemeasurement=ee.enum.exposemeasurement.hidden
      settings: SourceProductBaseCode=PS  InternalSimscapePortConfiguration="{\"Bottom\":[],\"Left\":[{\"id\":\"p\",\"label\":\"\",\"type\":\"foundation.electrical.electrical\"}],\"Right\":[{\"id\":\"n\",\"label\":\"\",\"type\":\"foundation.electrical.electrical\"}],\"Top\":[]}"
  Voltage-Current Simscape Interface (gnd){,1..5} (6 alike) : powerlib/Interface Elements/Voltage-Current Simscape Interface (gnd)  DFT=off  Fmode=Low pass filter (continuous)  T=1e-6  Ts=50e-6  i0=0  v0=0  Sd=Specialized Power Systems side  Measurements=off
      settings: SourceProductBaseCode=PS
  sps1 : PMIOPort  Side=Left
  sps3 : PMIOPort  Port=2  Side=Left
  sps5 : PMIOPort  Port=3  Side=Left
  sps : PMIOPort  Port=4  Side=Right
  sps2 : PMIOPort  Port=5  Side=Right
  sps4 : PMIOPort  Port=6  Side=Right
  connections:
  Voltage-Current Simscape Interface (gnd)5/RConn1 -- Fuse2/RConn1
  Voltage-Current Simscape Interface (gnd)4/RConn1 -- Fuse2/LConn1
  sps3/RConn1 -- Voltage-Current Simscape Interface (gnd)2/LConn1
  Voltage-Current Simscape Interface (gnd)/RConn1 -- Fuse/LConn1
  Voltage-Current Simscape Interface (gnd)/LConn1 -- sps1/RConn1
  Voltage-Current Simscape Interface (gnd)1/RConn1 -- Fuse/RConn1
  Voltage-Current Simscape Interface (gnd)2/RConn1 -- Fuse1/LConn1
  sps5/RConn1 -- Voltage-Current Simscape Interface (gnd)4/LConn1
  Voltage-Current Simscape Interface (gnd)5/LConn1 -- sps4/RConn1
  Voltage-Current Simscape Interface (gnd)3/RConn1 -- Fuse1/RConn1
  Voltage-Current Simscape Interface (gnd)1/LConn1 -- sps/RConn1
  Voltage-Current Simscape Interface (gnd)3/LConn1 -- sps2/RConn1

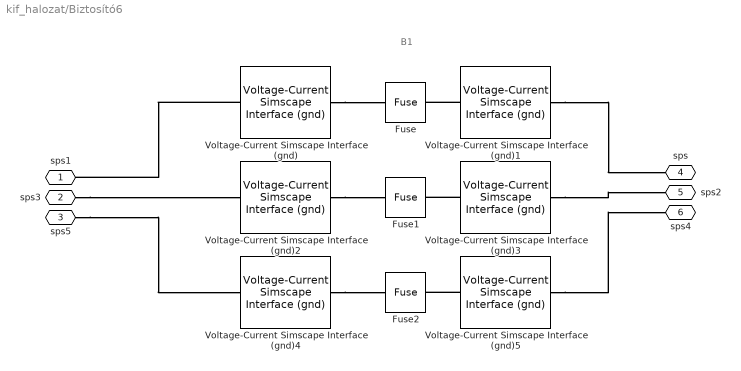
== system kif_halozat/Biztosító6 ==
  note: B1
  Fuse : ee_lib/Switches & Breakers/Fuse  prm=1  I_rated=125 A  melt_margin=1  T_fuse=0 s  I2t=1 s*A^2  I_vec=[1.9, 2, 2.5, 30] A  t_vec=[10000, 1, .3, .001] s  R_closed=0.01 Ohm  G_open=1e-8 1/Ohm  exposemeasurement=ee.enum.exposemeasurement.hidden
      settings: SourceProductBaseCode=PS  InternalSimscapePortConfiguration="{\"Bottom\":[],\"Left\":[{\"id\":\"p\",\"label\":\"\",\"type\":\"foundation.electrical.electrical\"}],\"Right\":[{\"id\":\"n\",\"label\":\"\",\"type\":\"foundation.electrical.electrical\"}],\"Top\":[]}"
  Fuse1 : ee_lib/Switches & Breakers/Fuse  prm=1  I_rated=125 A  melt_margin=1  T_fuse=0 s  I2t=1 s*A^2  I_vec=[1.9, 2, 2.5, 30] A  t_vec=[10000, 1, .3, .001] s  R_closed=0.01 Ohm  G_open=1e-8 1/Ohm  exposemeasurement=ee.enum.exposemeasurement.hidden
      settings: SourceProductBaseCode=PS  InternalSimscapePortConfiguration="{\"Bottom\":[],\"Left\":[{\"id\":\"p\",\"label\":\"\",\"type\":\"foundation.electrical.electrical\"}],\"Right\":[{\"id\":\"n\",\"label\":\"\",\"type\":\"foundation.electrical.electrical\"}],\"Top\":[]}"
  Fuse2 : ee_lib/Switches & Breakers/Fuse  prm=1  I_rated=125 A  melt_margin=1  T_fuse=0 s  I2t=1 s*A^2  I_vec=[1.9, 2, 2.5, 30] A  t_vec=[10000, 1, .3, .001] s  R_closed=0.01 Ohm  G_open=1e-8 1/Ohm  exposemeasurement=ee.enum.exposemeasurement.hidden
      settings: SourceProductBaseCode=PS  InternalSimscapePortConfiguration="{\"Bottom\":[],\"Left\":[{\"id\":\"p\",\"label\":\"\",\"type\":\"foundation.electrical.electrical\"}],\"Right\":[{\"id\":\"n\",\"label\":\"\",\"type\":\"foundation.electrical.electrical\"}],\"Top\":[]}"
  Voltage-Current Simscape Interface (gnd){,1..5} (6 alike) : powerlib/Interface Elements/Voltage-Current Simscape Interface (gnd)  DFT=off  Fmode=Low pass filter (continuous)  T=1e-6  Ts=50e-6  i0=0  v0=0  Sd=Specialized Power Systems side  Measurements=off
      settings: SourceProductBaseCode=PS
  sps1 : PMIOPort  Side=Left
  sps3 : PMIOPort  Port=2  Side=Left
  sps5 : PMIOPort  Port=3  Side=Left
  sps : PMIOPort  Port=4  Side=Right
  sps2 : PMIOPort  Port=5  Side=Right
  sps4 : PMIOPort  Port=6  Side=Right
  connections:
  Voltage-Current Simscape Interface (gnd)5/RConn1 -- Fuse2/RConn1
  Voltage-Current Simscape Interface (gnd)4/RConn1 -- Fuse2/LConn1
  sps3/RConn1 -- Voltage-Current Simscape Interface (gnd)2/LConn1
  Voltage-Current Simscape Interface (gnd)/RConn1 -- Fuse/LConn1
  Voltage-Current Simscape Interface (gnd)/LConn1 -- sps1/RConn1
  Voltage-Current Simscape Interface (gnd)1/RConn1 -- Fuse/RConn1
  Voltage-Current Simscape Interface (gnd)2/RConn1 -- Fuse1/LConn1
  sps5/RConn1 -- Voltage-Current Simscape Interface (gnd)4/LConn1
  Voltage-Current Simscape Interface (gnd)5/LConn1 -- sps4/RConn1
  Voltage-Current Simscape Interface (gnd)3/RConn1 -- Fuse1/RConn1
  Voltage-Current Simscape Interface (gnd)1/LConn1 -- sps/RConn1
  Voltage-Current Simscape Interface (gnd)3/LConn1 -- sps2/RConn1

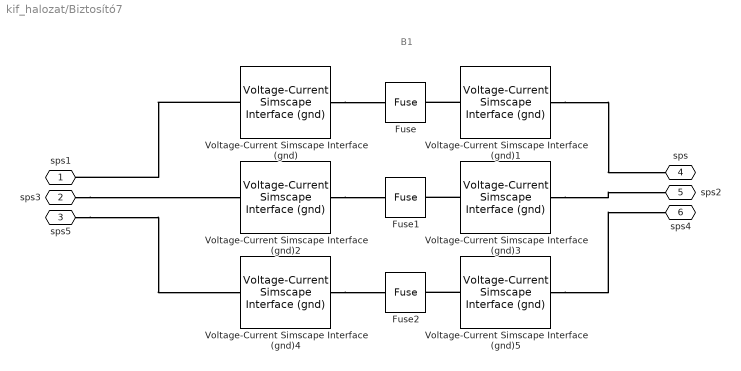
== system kif_halozat/Biztosító7 ==
  note: B1
  Fuse : ee_lib/Switches & Breakers/Fuse  prm=1  I_rated=125 A  melt_margin=1  T_fuse=0 s  I2t=1 s*A^2  I_vec=[1.9, 2, 2.5, 30] A  t_vec=[10000, 1, .3, .001] s  R_closed=0.01 Ohm  G_open=1e-8 1/Ohm  exposemeasurement=ee.enum.exposemeasurement.hidden
      settings: SourceProductBaseCode=PS  InternalSimscapePortConfiguration="{\"Bottom\":[],\"Left\":[{\"id\":\"p\",\"label\":\"\",\"type\":\"foundation.electrical.electrical\"}],\"Right\":[{\"id\":\"n\",\"label\":\"\",\"type\":\"foundation.electrical.electrical\"}],\"Top\":[]}"
  Fuse1 : ee_lib/Switches & Breakers/Fuse  prm=1  I_rated=125 A  melt_margin=1  T_fuse=0 s  I2t=1 s*A^2  I_vec=[1.9, 2, 2.5, 30] A  t_vec=[10000, 1, .3, .001] s  R_closed=0.01 Ohm  G_open=1e-8 1/Ohm  exposemeasurement=ee.enum.exposemeasurement.hidden
      settings: SourceProductBaseCode=PS  InternalSimscapePortConfiguration="{\"Bottom\":[],\"Left\":[{\"id\":\"p\",\"label\":\"\",\"type\":\"foundation.electrical.electrical\"}],\"Right\":[{\"id\":\"n\",\"label\":\"\",\"type\":\"foundation.electrical.electrical\"}],\"Top\":[]}"
  Fuse2 : ee_lib/Switches & Breakers/Fuse  prm=1  I_rated=125 A  melt_margin=1  T_fuse=0 s  I2t=1 s*A^2  I_vec=[1.9, 2, 2.5, 30] A  t_vec=[10000, 1, .3, .001] s  R_closed=0.01 Ohm  G_open=1e-8 1/Ohm  exposemeasurement=ee.enum.exposemeasurement.hidden
      settings: SourceProductBaseCode=PS  InternalSimscapePortConfiguration="{\"Bottom\":[],\"Left\":[{\"id\":\"p\",\"label\":\"\",\"type\":\"foundation.electrical.electrical\"}],\"Right\":[{\"id\":\"n\",\"label\":\"\",\"type\":\"foundation.electrical.electrical\"}],\"Top\":[]}"
  Voltage-Current Simscape Interface (gnd){,1..5} (6 alike) : powerlib/Interface Elements/Voltage-Current Simscape Interface (gnd)  DFT=off  Fmode=Low pass filter (continuous)  T=1e-6  Ts=50e-6  i0=0  v0=0  Sd=Specialized Power Systems side  Measurements=off
      settings: SourceProductBaseCode=PS
  sps1 : PMIOPort  Side=Left
  sps3 : PMIOPort  Port=2  Side=Left
  sps5 : PMIOPort  Port=3  Side=Left
  sps : PMIOPort  Port=4  Side=Right
  sps2 : PMIOPort  Port=5  Side=Right
  sps4 : PMIOPort  Port=6  Side=Right
  connections:
  Voltage-Current Simscape Interface (gnd)3/LConn1 -- sps2/RConn1
  Voltage-Current Simscape Interface (gnd)1/LConn1 -- sps/RConn1
  Voltage-Current Simscape Interface (gnd)3/RConn1 -- Fuse1/RConn1
  Voltage-Current Simscape Interface (gnd)5/LConn1 -- sps4/RConn1
  sps5/RConn1 -- Voltage-Current Simscape Interface (gnd)4/LConn1
  Voltage-Current Simscape Interface (gnd)2/RConn1 -- Fuse1/LConn1
  Voltage-Current Simscape Interface (gnd)1/RConn1 -- Fuse/RConn1
  Voltage-Current Simscape Interface (gnd)/LConn1 -- sps1/RConn1
  Voltage-Current Simscape Interface (gnd)/RConn1 -- Fuse/LConn1
  sps3/RConn1 -- Voltage-Current Simscape Interface (gnd)2/LConn1
  Voltage-Current Simscape Interface (gnd)4/RConn1 -- Fuse2/LConn1
  Voltage-Current Simscape Interface (gnd)5/RConn1 -- Fuse2/RConn1

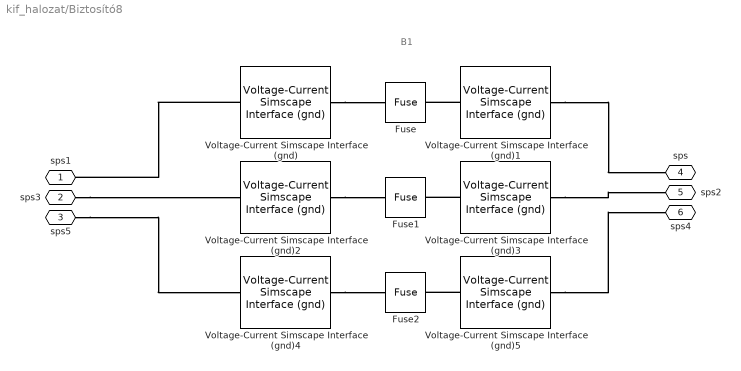
== system kif_halozat/Biztosító8 ==
  note: B1
  Fuse : ee_lib/Switches & Breakers/Fuse  prm=1  I_rated=125 A  melt_margin=1  T_fuse=0 s  I2t=1 s*A^2  I_vec=[1.9, 2, 2.5, 30] A  t_vec=[10000, 1, .3, .001] s  R_closed=0.01 Ohm  G_open=1e-8 1/Ohm  exposemeasurement=ee.enum.exposemeasurement.hidden
      settings: SourceProductBaseCode=PS  InternalSimscapePortConfiguration="{\"Bottom\":[],\"Left\":[{\"id\":\"p\",\"label\":\"\",\"type\":\"foundation.electrical.electrical\"}],\"Right\":[{\"id\":\"n\",\"label\":\"\",\"type\":\"foundation.electrical.electrical\"}],\"Top\":[]}"
  Fuse1 : ee_lib/Switches & Breakers/Fuse  prm=1  I_rated=125 A  melt_margin=1  T_fuse=0 s  I2t=1 s*A^2  I_vec=[1.9, 2, 2.5, 30] A  t_vec=[10000, 1, .3, .001] s  R_closed=0.01 Ohm  G_open=1e-8 1/Ohm  exposemeasurement=ee.enum.exposemeasurement.hidden
      settings: SourceProductBaseCode=PS  InternalSimscapePortConfiguration="{\"Bottom\":[],\"Left\":[{\"id\":\"p\",\"label\":\"\",\"type\":\"foundation.electrical.electrical\"}],\"Right\":[{\"id\":\"n\",\"label\":\"\",\"type\":\"foundation.electrical.electrical\"}],\"Top\":[]}"
  Fuse2 : ee_lib/Switches & Breakers/Fuse  prm=1  I_rated=125 A  melt_margin=1  T_fuse=0 s  I2t=1 s*A^2  I_vec=[1.9, 2, 2.5, 30] A  t_vec=[10000, 1, .3, .001] s  R_closed=0.01 Ohm  G_open=1e-8 1/Ohm  exposemeasurement=ee.enum.exposemeasurement.hidden
      settings: SourceProductBaseCode=PS  InternalSimscapePortConfiguration="{\"Bottom\":[],\"Left\":[{\"id\":\"p\",\"label\":\"\",\"type\":\"foundation.electrical.electrical\"}],\"Right\":[{\"id\":\"n\",\"label\":\"\",\"type\":\"foundation.electrical.electrical\"}],\"Top\":[]}"
  Voltage-Current Simscape Interface (gnd){,1..5} (6 alike) : powerlib/Interface Elements/Voltage-Current Simscape Interface (gnd)  DFT=off  Fmode=Low pass filter (continuous)  T=1e-6  Ts=50e-6  i0=0  v0=0  Sd=Specialized Power Systems side  Measurements=off
      settings: SourceProductBaseCode=PS
  sps1 : PMIOPort  Side=Left
  sps3 : PMIOPort  Port=2  Side=Left
  sps5 : PMIOPort  Port=3  Side=Left
  sps : PMIOPort  Port=4  Side=Right
  sps2 : PMIOPort  Port=5  Side=Right
  sps4 : PMIOPort  Port=6  Side=Right
  connections:
  Voltage-Current Simscape Interface (gnd)5/RConn1 -- Fuse2/RConn1
  Voltage-Current Simscape Interface (gnd)4/RConn1 -- Fuse2/LConn1
  sps3/RConn1 -- Voltage-Current Simscape Interface (gnd)2/LConn1
  Voltage-Current Simscape Interface (gnd)/RConn1 -- Fuse/LConn1
  Voltage-Current Simscape Interface (gnd)/LConn1 -- sps1/RConn1
  Voltage-Current Simscape Interface (gnd)1/RConn1 -- Fuse/RConn1
  Voltage-Current Simscape Interface (gnd)2/RConn1 -- Fuse1/LConn1
  sps5/RConn1 -- Voltage-Current Simscape Interface (gnd)4/LConn1
  Voltage-Current Simscape Interface (gnd)5/LConn1 -- sps4/RConn1
  Voltage-Current Simscape Interface (gnd)3/RConn1 -- Fuse1/RConn1
  Voltage-Current Simscape Interface (gnd)1/LConn1 -- sps/RConn1
  Voltage-Current Simscape Interface (gnd)3/LConn1 -- sps2/RConn1

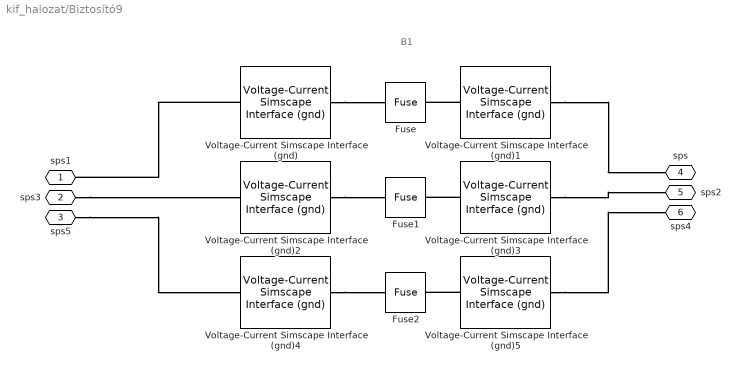
== system kif_halozat/Biztosító9 ==
  note: B1
  Fuse : ee_lib/Switches & Breakers/Fuse  prm=1  I_rated=125 A  melt_margin=1  T_fuse=0 s  I2t=1 s*A^2  I_vec=[1.9, 2, 2.5, 30] A  t_vec=[10000, 1, .3, .001] s  R_closed=0.01 Ohm  G_open=1e-8 1/Ohm  exposemeasurement=ee.enum.exposemeasurement.hidden
      settings: SourceProductBaseCode=PS  InternalSimscapePortConfiguration="{\"Bottom\":[],\"Left\":[{\"id\":\"p\",\"label\":\"\",\"type\":\"foundation.electrical.electrical\"}],\"Right\":[{\"id\":\"n\",\"label\":\"\",\"type\":\"foundation.electrical.electrical\"}],\"Top\":[]}"
  Fuse1 : ee_lib/Switches & Breakers/Fuse  prm=1  I_rated=125 A  melt_margin=1  T_fuse=0 s  I2t=1 s*A^2  I_vec=[1.9, 2, 2.5, 30] A  t_vec=[10000, 1, .3, .001] s  R_closed=0.01 Ohm  G_open=1e-8 1/Ohm  exposemeasurement=ee.enum.exposemeasurement.hidden
      settings: SourceProductBaseCode=PS  InternalSimscapePortConfiguration="{\"Bottom\":[],\"Left\":[{\"id\":\"p\",\"label\":\"\",\"type\":\"foundation.electrical.electrical\"}],\"Right\":[{\"id\":\"n\",\"label\":\"\",\"type\":\"foundation.electrical.electrical\"}],\"Top\":[]}"
  Fuse2 : ee_lib/Switches & Breakers/Fuse  prm=1  I_rated=125 A  melt_margin=1  T_fuse=0 s  I2t=1 s*A^2  I_vec=[1.9, 2, 2.5, 30] A  t_vec=[10000, 1, .3, .001] s  R_closed=0.01 Ohm  G_open=1e-8 1/Ohm  exposemeasurement=ee.enum.exposemeasurement.hidden
      settings: SourceProductBaseCode=PS  InternalSimscapePortConfiguration="{\"Bottom\":[],\"Left\":[{\"id\":\"p\",\"label\":\"\",\"type\":\"foundation.electrical.electrical\"}],\"Right\":[{\"id\":\"n\",\"label\":\"\",\"type\":\"foundation.electrical.electrical\"}],\"Top\":[]}"
  Voltage-Current Simscape Interface (gnd){,1..5} (6 alike) : powerlib/Interface Elements/Voltage-Current Simscape Interface (gnd)  DFT=off  Fmode=Low pass filter (continuous)  T=1e-6  Ts=50e-6  i0=0  v0=0  Sd=Specialized Power Systems side  Measurements=off
      settings: SourceProductBaseCode=PS
  sps1 : PMIOPort  Side=Left
  sps3 : PMIOPort  Port=2  Side=Left
  sps5 : PMIOPort  Port=3  Side=Left
  sps : PMIOPort  Port=4  Side=Right
  sps2 : PMIOPort  Port=5  Side=Right
  sps4 : PMIOPort  Port=6  Side=Right
  connections:
  Voltage-Current Simscape Interface (gnd)3/LConn1 -- sps2/RConn1
  Voltage-Current Simscape Interface (gnd)1/LConn1 -- sps/RConn1
  Voltage-Current Simscape Interface (gnd)3/RConn1 -- Fuse1/RConn1
  Voltage-Current Simscape Interface (gnd)5/LConn1 -- sps4/RConn1
  sps5/RConn1 -- Voltage-Current Simscape Interface (gnd)4/LConn1
  Voltage-Current Simscape Interface (gnd)2/RConn1 -- Fuse1/LConn1
  Voltage-Current Simscape Interface (gnd)1/RConn1 -- Fuse/RConn1
  Voltage-Current Simscape Interface (gnd)/LConn1 -- sps1/RConn1
  Voltage-Current Simscape Interface (gnd)/RConn1 -- Fuse/LConn1
  sps3/RConn1 -- Voltage-Current Simscape Interface (gnd)2/LConn1
  Voltage-Current Simscape Interface (gnd)4/RConn1 -- Fuse2/LConn1
  Voltage-Current Simscape Interface (gnd)5/RConn1 -- Fuse2/RConn1
